simulink model "Irrigation_Control_System_R2020a_CodeGeneration"  (R2020a)
settings: Solver=VariableStepAuto  StartTime=0.0  StopTime=10.0  RelTol=1e-3
settings Model: Creator=hp  LastModifiedBy=hp
settings DebuggingCC: UnconnectedInputMsg=none  UnconnectedOutputMsg=none  UnconnectedLineMsg=none
settings ModelReferenceCC: EnableRefExpFcnMdlSchedulingChecks=off
settings RTWCC: Description=Generic Real-Time Target

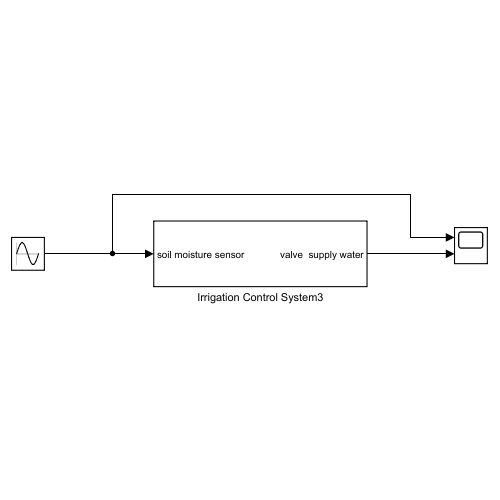
[thumbnail: Simulink's stored preview of the top-level diagram]
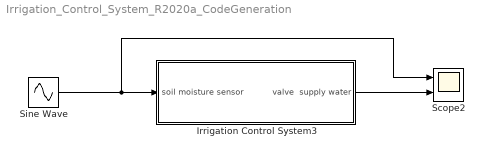
== system Irrigation_Control_System_R2020a_CodeGeneration ==
  Irrigation Control System3 : Subsystem
  Scope2 : Scope  NumInputPorts=2
  Sine Wave : Sin  Amplitude=50  SampleTime=0
  wires:
  Sine Wave/1 -> Irrigation Control System3/1(soil moisture sensor), Scope2/1
  Irrigation Control System3/1(valve  supply water) -> Scope2/2

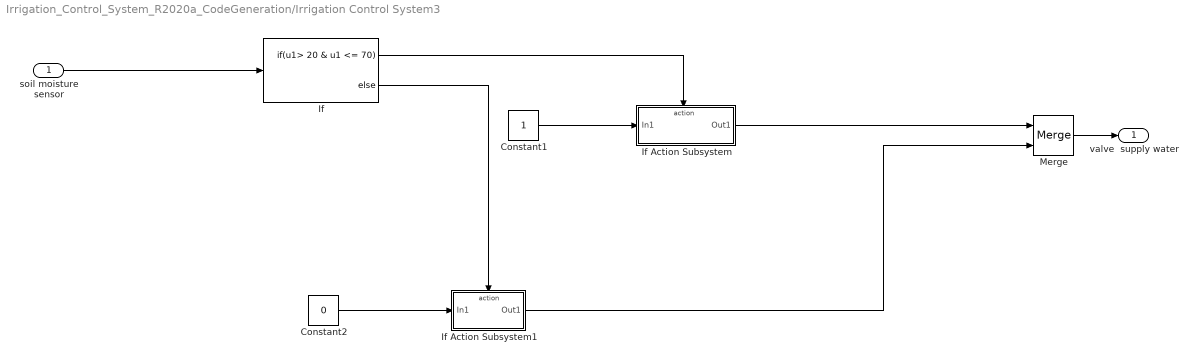
== system Irrigation_Control_System_R2020a_CodeGeneration/Irrigation Control System3 ==
  soil moisture sensor : Inport
  Constant1 : Constant
  Constant2 : Constant  Value=0
  If : If  IfExpression=u1> 20 & u1 <= 70
  If Action Subsystem : Subsystem  TreatAsAtomicUnit=on
  If Action Subsystem1 : Subsystem  TreatAsAtomicUnit=on
  Merge : Merge
  valve  supply water : Outport
  wires:
  If Action Subsystem1/1(Out1) -> Merge/2
  Constant1/1 -> If Action Subsystem/1(In1)
  Merge/1 -> valve  supply water/1
  soil moisture sensor/1 -> If/1
  If/1 -> If Action Subsystem/Action
  If/2 -> If Action Subsystem1/Action
  Constant2/1 -> If Action Subsystem1/1(In1)
  If Action Subsystem/1(Out1) -> Merge/1

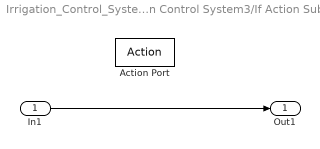
== system Irrigation_Control_System_R2020a_CodeGeneration/Irrigation Control System3/If Action Subsystem ==
  In1 : Inport
  Action Port : ActionPort
  Out1 : Outport
  wires:
  In1/1 -> Out1/1

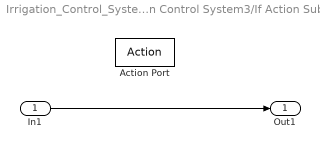
== system Irrigation_Control_System_R2020a_CodeGeneration/Irrigation Control System3/If Action Subsystem1 ==
  In1 : Inport
  Action Port : ActionPort
  Out1 : Outport
  wires:
  In1/1 -> Out1/1
